simulink model "swingup"  (Simulink 5.0)
settings: Solver=ode1  SolverMode=SingleTasking  StartTime=0.0  StopTime=inf  FixedStep=0.005  RelTol=1e-3
settings Model: LastModifiedBy=Administrator  ExtModeMexFile=rtwinext  ExtModeTrigDuration=100000  SimulationMode=external  LimitDataPoints=off  MaxDataPoints=20000  RTWSystemTargetFile=rtwin.tlc  RTWTemplateMakefile=rtwintmf  RTWOptions="-aCCOptimize=1 -aEnforceIntegerDowncast=1 -aExtMode=1 -aFoldNonRolledExpr=1 -aForceParamTrailComments=0 -aGenerateComments=1 -aGenerateReport=0 -aIncDataTypeInIds=0 -aIncHierarchyInIds=0 -aInlineInvariantSignals=0 -aInlineParameters=0 -aInlinedPrmAccess=\"Literals\" -aLocalBlockOutputs=1 -aMaxRTWIdLen=31 -aPrefixModelToSubsysFcnNames=1 -aRTWVerbose=1 -aRebuildAll=0 -aRollThreshold=5 -aShowEliminatedStatements=0"

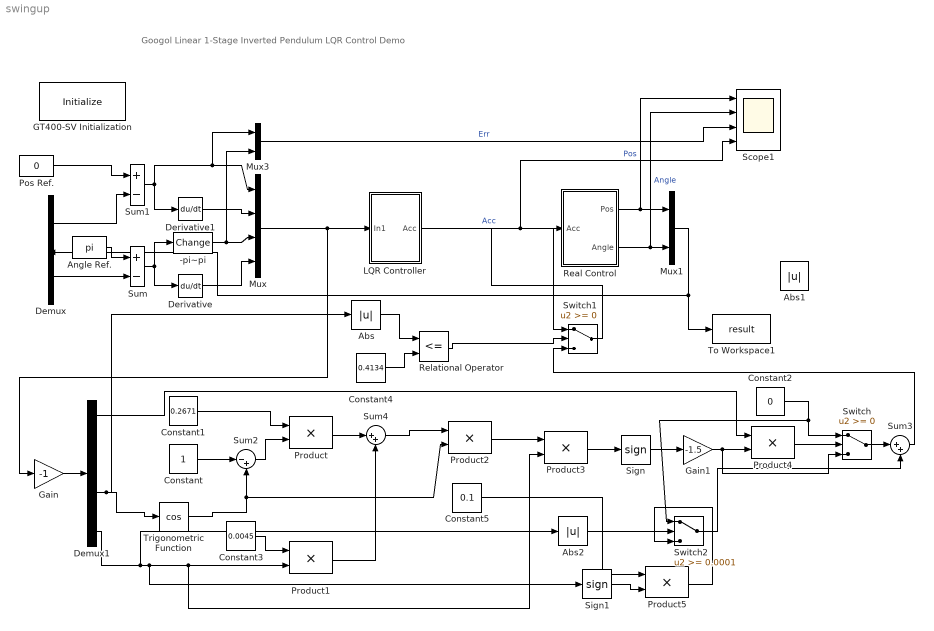
== system swingup ==
  note: Googol Linear 1-Stage Inverted Pendulum LQR Control Demo
  " -pi~pi" : S-Function  FunctionName=Change
      mask Type: Change
      mask Description:
      | Change input signal between -pi and pi in 2*pi period.
      | Block input:
      |     any double.
      | Block output:
      |     between -pi and pi.
      | eg:
      |     If input is 1.5*pi, then output is -0.5*pi.
      mask Help:
      | This block, "change", input signal between -pi and pi in 2*pi period.
      | Block input:
      |     any double.
      | Block output:
      |     between -pi and pi.
      | eg:
      |     input is 1.5*pi, then output is -0.5*pi.
      mask Display: plot([0:0.01:2*pi],sin([0:0.01:2*pi]));
  Abs : Abs  SaturateOnIntegerOverflow=on
  Abs1 : Abs  SaturateOnIntegerOverflow=on
  Abs2 : Abs  SaturateOnIntegerOverflow=on
  Angle Ref. : Constant  Value=pi
  Constant : Constant
  Constant1 : Constant  Value=0.2671
  Constant2 : Constant  Value=0
  Constant3 : Constant  Value=0.0045
  Constant4 : Constant  Value=0.4134
  Constant5 : Constant  Value=0.1
  Demux : Demux  Outputs=2
  Demux1 : Demux
  Derivative : Derivative
  Derivative1 : Derivative
  GT400-SV Initialization : S-Function  Priority=0  FunctionName=Initialize  Parameters=openloop  mask(Initialize){openloop=0}
      mask prompts: openloop "Control loop:"
      mask help:
      | Initializing the googol GT400-SV motion control board.
      | Block parameter:
      |     Control loop:
      |          0: closed-loop control.
      |          1: opened-loop control.
      mask Help: This initialize block initializes the googol GT400-SV motion control board.
      mask Display: disp('Initialize \nGT400-SV');
  Gain : Gain  Gain=-1  SaturateOnIntegerOverflow=on
  Gain1 : Gain  Gain=-1.5  SaturateOnIntegerOverflow=on
  LQR Controller : Subsystem  mask{x=-36.51, xdot=-23.62, angle=87.97, angledot=16.08}
      mask prompts: x "Kx"; xdot "Kx'"; angle "Ka"; angledot "Ka'"
  Mux : Mux
  Mux1 : Mux  Inputs=2
  Mux3 : Mux  Inputs=2
  Pos Ref. : Constant  Value=0
  Product{,1..5} (6 alike) : Product  SaturateOnIntegerOverflow=on
  Real Control : Subsystem
  Relational Operator : RelationalOperator  Operator=<=
  Scope1 : Scope  NumInputPorts=4
      settings: TickLabels=on  TimeRange=100  YMin=-0.00075~0~-0.5~-1  YMax=0.001~0.00275~3.5~1  SaveName=PosData  MaxDataPoints=20000
  Sign : Signum
  Sign1 : Signum
  Sum : Sum  Inputs=+-  SaturateOnIntegerOverflow=on
  Sum1 : Sum  Inputs=+-  SaturateOnIntegerOverflow=on
  Sum2 : Sum  Inputs=|-+  SaturateOnIntegerOverflow=on
  Sum3 : Sum  Inputs=|++  SaturateOnIntegerOverflow=on
  Sum4 : Sum  Inputs=|++  SaturateOnIntegerOverflow=on
  Switch : Switch  SaturateOnIntegerOverflow=on
  Switch1 : Switch  SaturateOnIntegerOverflow=on
  Switch2 : Switch  Threshold=0.0001  ShowAdditionalParam=on  SaturateOnIntegerOverflow=on
  To Workspace1 : ToWorkspace  VariableName=result  SampleTime=0.005  SaveFormat=Array
  Trigonometric Function : Trigonometry  Operator=cos
  wires:
  Mux/1 -> LQR Controller/1(In1), Gain/1
  Mux1/1 -> Demux/1, To Workspace1/1
  Sum/1 -> Derivative/1, " -pi~pi"/1
  Demux/2 -> Sum/2
  Demux/1 -> Sum1/2
  Sum1/1 -> Derivative1/1, Mux/1, Mux3/1
  Real Control/2(Angle) -> Mux1/2, Scope1/2  "Angle"
  Angle Ref./1 -> Sum/1
  " -pi~pi"/1 -> Mux/3, Mux3/2
  Real Control/1(Pos) -> Mux1/1, Scope1/1  "Pos"
  Derivative/1 -> Mux/4
  Derivative1/1 -> Mux/2
  Mux3/1 -> Scope1/3  "Err"
  Pos Ref./1 -> Sum1/1
  Constant1/1 -> Product/1
  Constant/1 -> Sum2/1
  Sum2/1 -> Product/2
  Trigonometric Function/1 -> Sum2/2, Product2/2
  Product1/1 -> Sum4/2
  Constant3/1 -> Product1/1
  Gain/1 -> Demux1/1
  Demux1/4 -> Abs2/1, Product1/2, Product3/2, Sign1/1
  Demux1/3 -> Abs/1, Trigonometric Function/1
  Sum4/1 -> Product2/1
  Product/1 -> Sum4/1
  Product2/1 -> Product3/1
  Product3/1 -> Sign/1
  Sign/1 -> Gain1/1
  Gain1/1 -> Product4/2, Switch/3
  Demux1/1 -> Product4/1
  Product4/1 -> Switch/2
  Constant2/1 -> Switch/1, Switch2/1
  Relational Operator/1 -> Switch1/2
  Abs/1 -> Relational Operator/1
  Constant4/1 -> Relational Operator/2
  LQR Controller/1(Acc) -> Switch1/1  "Acc"
  Switch1/1 -> Real Control/1(Acc), Scope1/4
  Switch/1 -> Sum3/1
  Sum3/1 -> Switch1/3
  Switch2/1 -> Sum3/2
  Abs2/1 -> Switch2/2
  Constant5/1 -> Product5/1
  Sign1/1 -> Product5/2
  Product5/1 -> Switch2/3

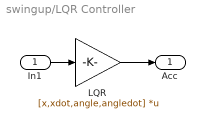
== system swingup/LQR Controller ==
  In1 : Inport
  LQR : Gain  Gain=[x,xdot,angle,angledot]  Multiplication=Matrix(K*u)  SaturateOnIntegerOverflow=on
  Acc : Outport
  wires:
  LQR/1 -> Acc/1
  In1/1 -> LQR/1

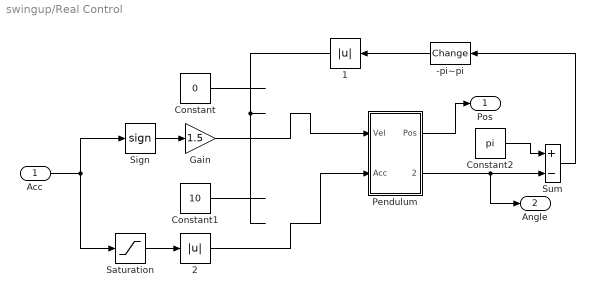
== system swingup/Real Control ==
  Acc : Inport
  " -pi~pi" : S-Function  Orientation=left  AncestorBlock=googolbox/GT-400-SV Block Library/ -pi~pi  FunctionName=Change
      mask Type: Change
      mask Description:
      | Change input signal between -pi and pi in 2*pi period.
      | Block input:
      |     any double.
      | Block output:
      |     between -pi and pi.
      | eg:
      |     If input is 1.5*pi, then output is -0.5*pi.
      mask Help:
      | This block, "change", input signal between -pi and pi in 2*pi period.
      | Block input:
      |     any double.
      | Block output:
      |     between -pi and pi.
      | eg:
      |     input is 1.5*pi, then output is -0.5*pi.
      mask Display: plot([0:0.01:2*pi],sin([0:0.01:2*pi]));
  " 1" : Abs  Orientation=left  SaturateOnIntegerOverflow=on
  " 2" : Abs  SaturateOnIntegerOverflow=on
  Constant : Constant  Value=0
  Constant1 : Constant  Value=10
  Constant2 : Constant  Value=pi
  Gain : Gain  Gain=1.5  SaturateOnIntegerOverflow=on
  Pendulum : Subsystem
  Saturation : Saturate  UpperLimit=15  LowerLimit=-15
  Sign : Signum
  Sum : Sum  Inputs=+-  SaturateOnIntegerOverflow=on
  Pos : Outport
  Angle : Outport  Port=2
  wires:
  Acc/1 -> Saturation/1, Sign/1
  Sign/1 -> Gain/1
  Pendulum/2(Angle) -> Angle/1, Sum/2
  Pendulum/1(Pos) -> Pos/1
  Saturation/1 -> " 2"/1
  " 1"/1 -> ?
  " -pi~pi"/1 -> " 1"/1
  Constant2/1 -> Sum/1
  Sum/1 -> " -pi~pi"/1
  Gain/1 -> Pendulum/1(Vel)
  Constant/1 -> ?
  " 2"/1 -> Pendulum/2(Acc)
  Constant1/1 -> ?

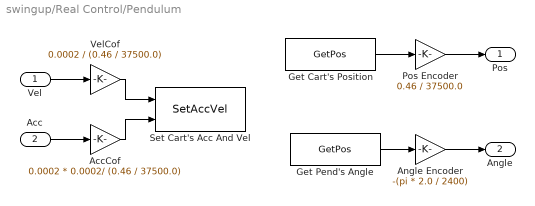
== system swingup/Real Control/Pendulum ==
  Vel : Inport
  Acc : Inport  Port=2
  AccCof : Gain  Gain=0.0002 * 0.0002/ (0.46 / 37500.0)  SaturateOnIntegerOverflow=on
  Angle Encoder : Gain  Gain=-(pi * 2.0 / 2400)  SaturateOnIntegerOverflow=on
  Get Cart's Position : S-Function  Priority=1  FunctionName=GetPos  Parameters=axis  mask(GetPos){axis=1}
      mask prompts: axis "Axis number:"
      mask help:
      | Getting the current axis position value in encoder' counts.
      | Block parameter:
      |     Axis number:  must be between 1 and 6, default is 1.
      | Block output:
      |     1~4: current axis' encoder reading counts.
      |     5/6: assistant encoder 1/2 reading counts.
      mask Help:
      | This block, GetPos, is intended for getting the current axis position value in encoder' counts. This value represents the actual position for the axis
      | at the current sample time. This command operates for all profile modes.
      | The value returned is a 32-bit signed number with units of counts.
      | The range is -1,073,741,824 to 1,073,741,823.
      | 
      | You can recalculate obtained value into meter units via multiplication by the scaler coefficient .
      | 
      | Block parameter:
      |     Axis number:  must be between 1 and 4, default is 1.
      | Block input: none.
      | Block output:
      |         1~4: current axis' encoder reading counts.
      |         5/6: assistant encoder 1/2 reading counts.
      mask Display:
      | disp('GetPos');
      | port_label('output', 1, 'Pos');
  Get Pend's Angle : S-Function  Priority=1  FunctionName=GetPos  Parameters=axis  mask(GetPos){axis=2}
      mask prompts: axis "Axis number:"
      mask help:
      | Getting the current axis position value in encoder' counts.
      | Block parameter:
      |     Axis number:  must be between 1 and 6, default is 1.
      | Block output:
      |     1~4: current axis' encoder reading counts.
      |     5/6: assistant encoder 1/2 reading counts.
      mask Help:
      | This block, GetPos, is intended for getting the current axis position value in encoder' counts. This value represents the actual position for the axis
      | at the current sample time. This command operates for all profile modes.
      | The value returned is a 32-bit signed number with units of counts.
      | The range is -1,073,741,824 to 1,073,741,823.
      | 
      | You can recalculate obtained value into meter units via multiplication by the scaler coefficient .
      | 
      | Block parameter:
      |     Axis number:  must be between 1 and 4, default is 1.
      | Block input: none.
      | Block output:
      |         1~4: current axis' encoder reading counts.
      |         5/6: assistant encoder 1/2 reading counts.
      mask Display:
      | disp('GetPos');
      | port_label('output', 1, 'Pos');
  Pos Encoder : Gain  Gain=0.46 / 37500.0  SaturateOnIntegerOverflow=on
  Set Cart's Acc And Vel : S-Function  Priority=1  FunctionName=SetAccVel  Parameters=axis, vel, pos  mask(SetAccVel){axis=1, vel=0.1, pos=250000}
      mask prompts: axis "Axis number:"; vel "Back velocity:"; pos "Back position:"
      mask help:
      | Setting the current axis' acceleration and velocity.
      |
      | Block parameter:
      |     Axis number:
      |         must be between 1 and 4, default is 1;
      |     Back velocity:
      |          After the current axis' limit reached, the moter will moves back as this  velocity, it must >=0;
      |     Back position:
      |          After the current axis' limit reached, the moter will moves back to this postion relative to limit, it must >=0;
      |
      | Block input:
      |     Vel: the current axis' velocity.
      |     Acc: the current axis' acceleration.
      mask Help:
      | This SetAccVel bolck Sets the current axis' acceleration and velocity.
      | Block parameter:
      |     Axis number: must be between 1 and 4, default is 1.
      | Block input:
      |     Vel: the current axis' velocity.
      |     Acc: the current axis' acceleration.
      mask Display:
      | disp('          SetAccVel');
      | port_label('input', 1, 'Vel');
      | port_label('input', 2, 'Acc');
  VelCof : Gain  Gain=0.0002 / (0.46 / 37500.0)  SaturateOnIntegerOverflow=on
  Pos : Outport
  Angle : Outport  Port=2
  wires:
  Get Cart's Position/1 -> Pos Encoder/1
  Vel/1 -> VelCof/1
  Acc/1 -> AccCof/1
  Get Pend's Angle/1 -> Angle Encoder/1
  Pos Encoder/1 -> Pos/1
  Angle Encoder/1 -> Angle/1
  VelCof/1 -> Set Cart's Acc And Vel/1
  AccCof/1 -> Set Cart's Acc And Vel/2
